simulink model "exercise_3b"  (R2018a)
settings: Solver=VariableStepAuto  StartTime=0.0  StopTime=10.0  RelTol=1e-3
undefined symbols (not defined in the file or in its folder): p
libraries: simulink x1
settings Model: Creator=mz-171742  LastModifiedBy=mz-171742

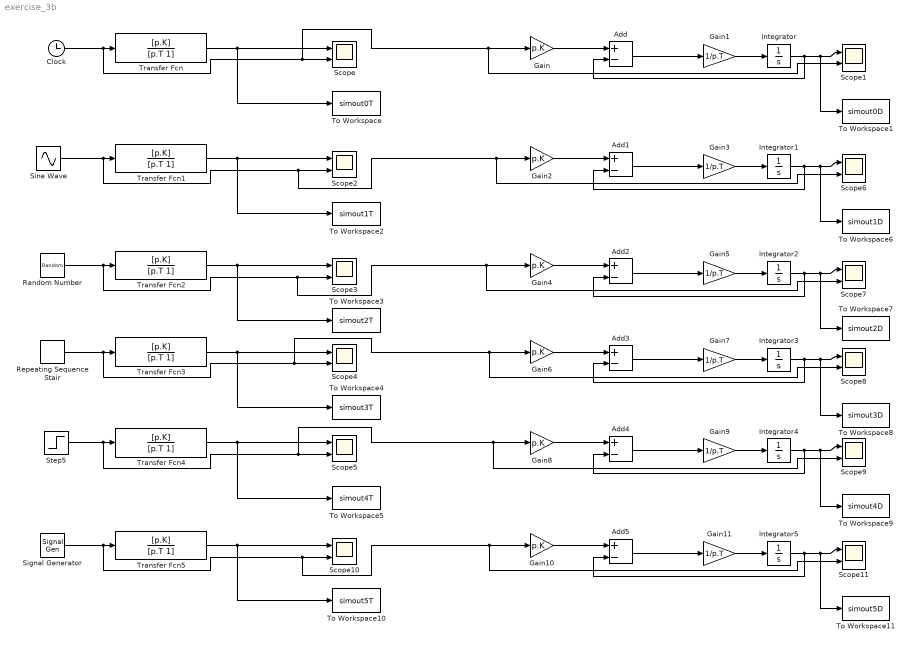
== system exercise_3b ==
  Add{,1..5} (6 alike) : Sum  Inputs=+-
  Clock : Clock
  Gain{,2,4,6,8,10} (6 alike) : Gain  Gain=p.K
  Gain{1,3,5,7,9,11} (6 alike) : Gain  Gain=1/p.T
  Integrator{,1..5} (6 alike) : Integrator
  Random Number : RandomNumber  SampleTime=0.1
  Repeating Sequence Stair : simulink/Sources/Repeating Sequence Stair  OutValues=[3 1 4 2 1].'  tsamp=-1  OutMin=[]  OutMax=[]  OutDataTypeStr=double  OutputDataTypeScalingMode=double  OutDataType=fixdt(0,8)  ConRadixGroup=Best Precision: Vector-wise  OutScaling=2^-12
  Scope{,1..11} (12 alike) : Scope  NumInputPorts=2
  Signal Generator : SignalGenerator  Units=rad/sec
  Sine Wave : Sin  SampleTime=0
  Step5 : Step  SampleTime=0
  To Workspace : ToWorkspace  VariableName=simout0T  SaveFormat=Structure With Time  SampleTime=-1
  To Workspace1 : ToWorkspace  VariableName=simout0D  SaveFormat=Structure With Time  SampleTime=-1
  To Workspace10 : ToWorkspace  VariableName=simout5T  SaveFormat=Structure With Time  SampleTime=-1
  To Workspace11 : ToWorkspace  VariableName=simout5D  SaveFormat=Structure With Time  SampleTime=-1
  To Workspace2 : ToWorkspace  VariableName=simout1T  SaveFormat=Structure With Time  SampleTime=-1
  To Workspace3 : ToWorkspace  VariableName=simout2T  SaveFormat=Structure With Time  SampleTime=-1
  To Workspace4 : ToWorkspace  VariableName=simout3T  SaveFormat=Structure With Time  SampleTime=-1
  To Workspace5 : ToWorkspace  VariableName=simout4T  SaveFormat=Structure With Time  SampleTime=-1
  To Workspace6 : ToWorkspace  VariableName=simout1D  SaveFormat=Structure With Time  SampleTime=-1
  To Workspace7 : ToWorkspace  VariableName=simout2D  SaveFormat=Structure With Time  SampleTime=-1
  To Workspace8 : ToWorkspace  VariableName=simout3D  SaveFormat=Structure With Time  SampleTime=-1
  To Workspace9 : ToWorkspace  VariableName=simout4D  SaveFormat=Structure With Time  SampleTime=-1
  Transfer Fcn{,1..5} (6 alike) : TransferFcn  Numerator=[p.K]  Denominator=[p.T 1]
  wires:
  Transfer Fcn/1 -> To Workspace/1, Scope/1
  Clock/1 -> Scope1/2, Gain/1, Scope/2, Transfer Fcn/1
  Gain/1 -> Add/1
  Add/1 -> Gain1/1
  Gain1/1 -> Integrator/1
  Integrator/1 -> Add/2, To Workspace1/1, Scope1/1
  Transfer Fcn1/1 -> To Workspace2/1, Scope2/1
  Transfer Fcn2/1 -> To Workspace3/1, Scope3/1
  Transfer Fcn3/1 -> To Workspace4/1, Scope4/1
  Transfer Fcn4/1 -> To Workspace5/1, Scope5/1
  Gain3/1 -> Integrator1/1
  Add1/1 -> Gain3/1
  Integrator1/1 -> Add1/2, To Workspace6/1, Scope6/1
  Gain2/1 -> Add1/1
  Sine Wave/1 -> Scope6/2, Gain2/1, Scope2/2, Transfer Fcn1/1
  Random Number/1 -> Scope7/2, Gain4/1, Scope3/2, Transfer Fcn2/1
  Gain4/1 -> Add2/1
  Integrator2/1 -> Add2/2, To Workspace7/1, Scope7/1
  Add2/1 -> Gain5/1
  Gain5/1 -> Integrator2/1
  Integrator3/1 -> Add3/2, To Workspace8/1, Scope8/1
  Add3/1 -> Gain7/1
  Gain7/1 -> Integrator3/1
  Gain6/1 -> Add3/1
  Repeating Sequence Stair/1 -> Scope8/2, Gain6/1, Scope4/2, Transfer Fcn3/1
  Add4/1 -> Gain9/1
  Integrator4/1 -> Add4/2, To Workspace9/1, Scope9/1
  Gain8/1 -> Add4/1
  Step5/1 -> Scope9/2, Gain8/1, Scope5/2, Transfer Fcn4/1
  Gain9/1 -> Integrator4/1
  Transfer Fcn5/1 -> To Workspace10/1, Scope10/1
  Signal Generator/1 -> Scope11/2, Gain10/1, Scope10/2, Transfer Fcn5/1
  Gain10/1 -> Add5/1
  Integrator5/1 -> Add5/2, To Workspace11/1, Scope11/1
  Gain11/1 -> Integrator5/1
  Add5/1 -> Gain11/1
